simulink model "mVarStep"  (Simulink 7.1)
settings: Solver=VariableStepDiscrete  StartTime=0.0  StopTime=10.0  MaxStep=0.2  RelTol=1e-3
settings Model: Creator=jcobleig  LastModifiedBy=jcobleig
settings OptimizationCC: InlineParams=on  InitFltsAndDblsToZero=off  EfficientMapNaN2IntZero=off
settings DebuggingCC: StrictBusMsg=ErrorOnBusTreatedAsVector

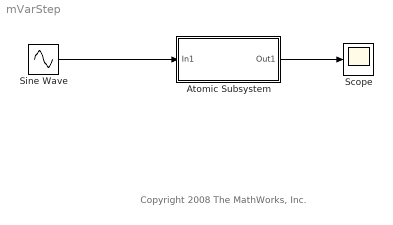
== system mVarStep ==
  note: Copyright 2008 The MathWorks, Inc.
  Atomic Subsystem : Subsystem  TreatAsAtomicUnit=on
  Scope : Scope
  Sine Wave : Sin  SampleTime=0
  wires:
  Sine Wave/1 -> Atomic Subsystem/1(In1)
  Atomic Subsystem/1(Out1) -> Scope/1

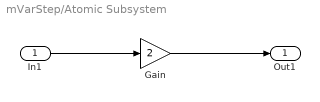
== system mVarStep/Atomic Subsystem ==
  In1 : Inport  OutDataType=sfix(16)  OutScaling=2^0
  Gain : Gain  Gain=2  ParameterDataType=sfix(16)  ParameterScaling=2^0  OutDataType=sfix(16)  OutScaling=2^0
  Out1 : Outport  OutDataType=sfix(16)  OutScaling=2^0
  wires:
  In1/1 -> Gain/1
  Gain/1 -> Out1/1
